simulink model "convertors"  (R2025a)
settings: Solver=VariableStepAuto  StartTime=0.0  StopTime=10.0  RelTol=1e-3
libraries: spsVoltageMeasurementLib x7, spsMosfetLib x6, spsThyristorLib x6, spsSeriesRLCBranchLib x5, spsACVoltageSourceLib x3, spsDCVoltageSourceLib x1, simulink x1, sps_lib x1
settings Model: Creator=gades  LastModifiedBy=gades

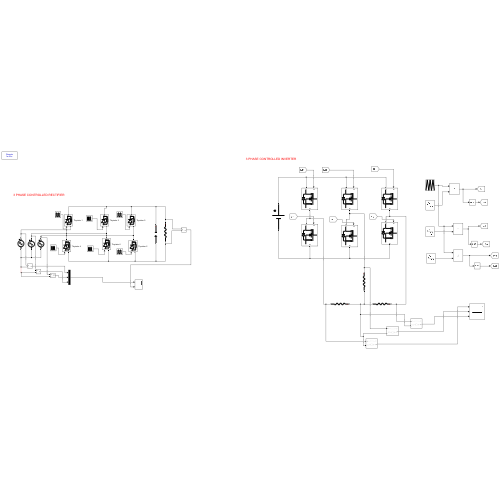
[thumbnail: Simulink's stored preview of the top-level diagram]
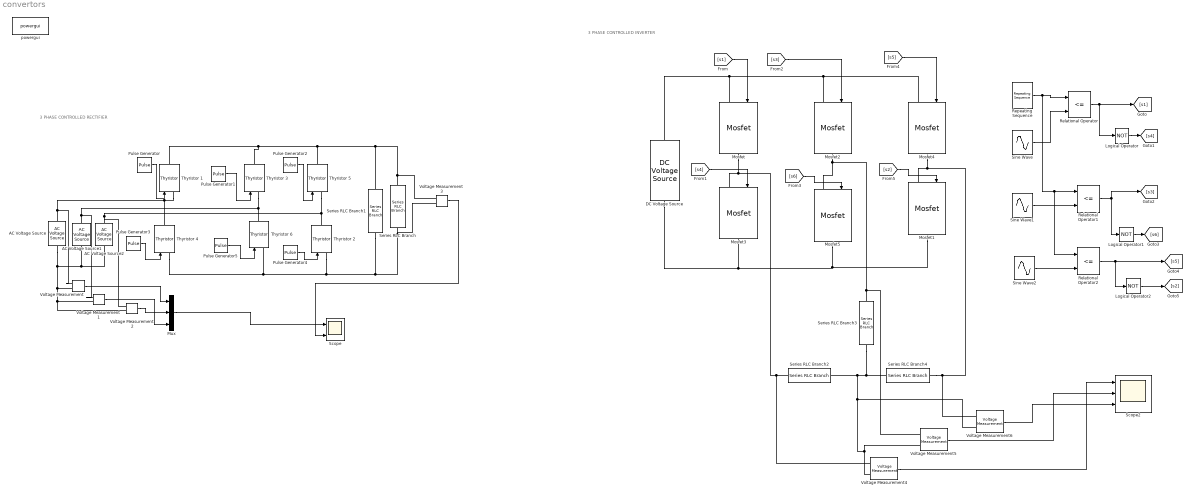
== system convertors ==
  note: 3 PHASE CONTROLLED INVERTER
  note: 3 PHASE CONTROLLED RECTIFIER
  AC Voltage Source : spsACVoltageSourceLib/AC Voltage Source  Amplitude=110  Phase=0  Frequency=50  SampleTime=0  Measurements=None  BusType=swing  Pref=10e3  Qref=0  Qmin=-inf  Qmax=+inf
  AC Voltage Source1 : spsACVoltageSourceLib/AC Voltage Source  Amplitude=110  Phase=-120  Frequency=50  SampleTime=0  Measurements=None  BusType=swing  Pref=10e3  Qref=0  Qmin=-inf  Qmax=+inf
  AC Voltage Source2 : spsACVoltageSourceLib/AC Voltage Source  Amplitude=110  Phase=+120  Frequency=50  SampleTime=0  Measurements=None  BusType=swing  Pref=10e3  Qref=0  Qmin=-inf  Qmax=+inf
  DC Voltage Source : spsDCVoltageSourceLib/DC Voltage Source  Amplitude=48  Measurements=None
  Logical Operator : Logic  Operator=NOT  AllPortsSameDT=off  OutDataTypeStr=boolean
  Logical Operator1 : Logic  Operator=NOT  AllPortsSameDT=off  OutDataTypeStr=boolean
  Logical Operator2 : Logic  Operator=NOT  AllPortsSameDT=off  OutDataTypeStr=boolean
  Mosfet{,1..5} (6 alike) : spsMosfetLib/Mosfet  Ron=0.1  Lon=0  Rd=0.01  Vfd=0  IC=0  Rs=1e5  Cs=inf  Measurements=off
  Mux : Mux  Inputs=3
  Pulse Generator : DiscretePulseGenerator  PulseType=Time based  Period=0.02  PulseWidth=(120/360)*100  PhaseDelay=(60/360)*0.02
  Pulse Generator1 : DiscretePulseGenerator  PulseType=Time based  Period=0.02  PulseWidth=(120/360)*100  PhaseDelay=(180/360)*0.02
  Pulse Generator2 : DiscretePulseGenerator  PulseType=Time based  Period=0.02  PulseWidth=(120/360)*100  PhaseDelay=(300/360)*0.02
  Pulse Generator3 : DiscretePulseGenerator  PulseType=Time based  Period=0.02  PulseWidth=(120/360)*100  PhaseDelay=(240/360)*0.02
  Pulse Generator4 : DiscretePulseGenerator  PulseType=Time based  Period=0.02  PulseWidth=(120/360)*100  PhaseDelay=(120/360)*0.02
  Pulse Generator5 : DiscretePulseGenerator  PulseType=Time based  Period=0.02  PulseWidth=(120/360)*100  PhaseDelay=(360/360)*0.02
  Relational Operator : RelationalOperator  Operator=<=  OutDataTypeStr=boolean  RndMeth=Simplest  InputSameDT=off
  Relational Operator1 : RelationalOperator  Operator=<=  OutDataTypeStr=boolean  RndMeth=Simplest  InputSameDT=off
  Relational Operator2 : RelationalOperator  Operator=<=  OutDataTypeStr=boolean  RndMeth=Simplest  InputSameDT=off
  Repeating Sequence : simulink/Sources/Repeating Sequence  rep_seq_t=[0 0.000005 0.00001]  rep_seq_y=[0 5 0]
  Scope : Scope  NumInputPorts=2
      settings: ActiveDisplayYMinimum=-137.5  ActiveDisplayYMaximum=137.5
  Scope2 : Scope  NumInputPorts=3
      settings: ActiveDisplayYMinimum=-39.603881972352511  ActiveDisplayYMaximum=39.603881972393324  DataLoggingVariableName=ScopeData2
  Series RLC Branch{,2..4} (4 alike) : spsSeriesRLCBranchLib/Series RLC Branch  LConnTagsString=__new0  RConnTagsString=__new0  BranchType=R  Resistance=10  Inductance=1e-3  SetiL0=off  InitialCurrent=0  Capacitance=1e-6  Setx0=off  InitialVoltage=0  Measurements=None
  Series RLC Branch1 : spsSeriesRLCBranchLib/Series RLC Branch  LConnTagsString=__new0  RConnTagsString=__new0  BranchType=C  Resistance=10  Inductance=1e-3  SetiL0=off  InitialCurrent=0  Capacitance=330e-3  Setx0=off  InitialVoltage=0  Measurements=None
  Sine Wave : Sin  Amplitude=5  Frequency=50*2*pi  SampleTime=0
  Sine Wave1 : Sin  Amplitude=5  Frequency=50*2*pi  Phase=(2*pi)/3  SampleTime=0
  Sine Wave2 : Sin  Amplitude=5  Frequency=50*2*pi  Phase=(4*pi)/3  SampleTime=0
  Thyristor {1..6} (6 alike) : spsThyristorLib/Thyristor  Ron=0.001  Lon=0  Vf=0.8  IC=0  Rs=500  Cs=250e-9  Measurements=off
  Voltage Measurement{,1..6} (7 alike) : spsVoltageMeasurementLib/Voltage Measurement  PhasorSimulation=off  OutputType=Complex  PSBequivalent=0
  powergui : sps_lib/powergui  Priority=1  SimulationMode=Discrete  SampleTime=1e-6  frequency=60  Iterations=50  frequencyindice=0  Pbase=100e6  ErrMax=1e-4  UnitsV=kV  UnitsW=MW  buscounter=0  FunctionMessages=off  echomessages=off  EnableUseOfTLC=off  CurrentSourceSwitches=off  DisableSnubberDevices=off  DisableRonSwitches=off  DisableVfSwitches=off  DisplayEquations=off  AutomaticDiscreteSolvers=off  SolverType=Tustin/Backward Euler (TBE)  Interpol=off  ExternalGateDelay=off  methode=off  Ts=100  x0status=blocks  SPID=on  SwTol=0  HookPort=off  NonlinearTolerance=1e-4  nMaxIteration=100  ContinueOnMaxIteration=off  RestoreLinks=warning  ResistiveCurrentMeasurement=off  Frange=[0:2:500]  Ylog=off  Xlog=on  ShowGrid=off  save=off  variable=ZData  structure=0  ZoomFFT=off  StartTime=0.0  cycles=1  DisplayStyle=1  fundamental=60  FreqAxis=off  MaxFrequency=1000  frequencyindicesteady=1  RmsSteady=1  display=off
  wires:
  Pulse Generator/1 -> Thyristor 1/1
  Pulse Generator1/1 -> Thyristor 3/1
  Pulse Generator2/1 -> Thyristor 5/1
  Pulse Generator3/1 -> Thyristor 4/1
  Pulse Generator4/1 -> Thyristor 2/1
  Voltage Measurement/1 -> Mux/1
  Voltage Measurement1/1 -> Mux/3
  Voltage Measurement2/1 -> Mux/2
  Mux/1 -> Scope/1
  Voltage Measurement3/1 -> Scope/2
  Pulse Generator5/1 -> Thyristor 6/1
  Voltage Measurement4/1 -> Scope2/1
  Voltage Measurement5/1 -> Scope2/2
  Sine Wave/1 -> Relational Operator/2
  Relational Operator/1 -> Logical Operator/1, [s1]
  [s1] -> Mosfet/1
  Logical Operator/1 -> [s4]
  [s4] -> Mosfet3/1
  Relational Operator1/1 -> [s3], Logical Operator1/1
  Logical Operator1/1 -> [s6]
  Sine Wave1/1 -> Relational Operator1/2
  [s3] -> Mosfet2/1
  [s6] -> Mosfet5/1
  [s5] -> Mosfet4/1
  [s2] -> Mosfet1/1
  Relational Operator2/1 -> Logical Operator2/1, [s5]
  Logical Operator2/1 -> [s2]
  Sine Wave2/1 -> Relational Operator2/2
  Repeating Sequence/1 -> Relational Operator2/1, Relational Operator1/1, Relational Operator/1
  Voltage Measurement6/1 -> Scope2/3
  connections:
  AC Voltage Source/LConn1 -- Voltage Measurement2/LConn2 -- Voltage Measurement1/LConn2 -- Voltage Measurement/LConn2 -- AC Voltage Source2/LConn1 -- AC Voltage Source1/LConn1
  Thyristor 1/LConn1 -- Voltage Measurement/LConn1 -- AC Voltage Source/RConn1 -- Thyristor 4/RConn1
  Thyristor 3/LConn1 -- Voltage Measurement1/LConn1 -- AC Voltage Source1/RConn1 -- Thyristor 6/RConn1
  Thyristor 5/LConn1 -- Voltage Measurement2/LConn1 -- AC Voltage Source2/RConn1 -- Thyristor 2/RConn1
  Thyristor 1/RConn1 -- Series RLC Branch1/LConn1 -- Voltage Measurement3/LConn1 -- Series RLC Branch/LConn1 -- Thyristor 5/RConn1 -- Thyristor 3/RConn1
  Thyristor 4/LConn1 -- Series RLC Branch1/RConn1 -- Voltage Measurement3/LConn2 -- Series RLC Branch/RConn1 -- Thyristor 2/LConn1 -- Thyristor 6/LConn1
  Mosfet/RConn1 -- Voltage Measurement4/LConn1 -- Series RLC Branch2/RConn1 -- Mosfet3/LConn1
  Mosfet2/RConn1 -- Voltage Measurement5/LConn1 -- Series RLC Branch3/LConn1 -- Mosfet5/LConn1
  Mosfet4/RConn1 -- Voltage Measurement6/LConn1 -- Series RLC Branch4/LConn1 -- Mosfet1/LConn1
  DC Voltage Source/LConn1 -- Mosfet1/RConn1 -- Mosfet5/RConn1 -- Mosfet3/RConn1
  DC Voltage Source/RConn1 -- Mosfet4/LConn1 -- Mosfet2/LConn1 -- Mosfet/LConn1
  Series RLC Branch3/RConn1 -- Voltage Measurement5/LConn2 -- Voltage Measurement4/LConn2 -- Voltage Measurement6/LConn2 -- Series RLC Branch2/LConn1 -- Series RLC Branch4/RConn1
